simulink model "trajectory_planner"  (R2019b)
settings: Solver=FixedStepAuto  StartTime=0.0  StopTime=10.0  RelTol=1e-3
undefined symbols (not defined in the file): v
libraries: robotcorelib x1
settings Model: Creator=logan  LastModifiedBy=logan
settings OptimizationCC: DefaultParameterBehavior=Inlined  UseDivisionForNetSlopeComputation=on  GainParamInheritBuiltInType=on  UseFloatMulNetSlope=on  InlineInvariantSignals=on  PassReuseOutputArgsAs=Individual arguments  ZeroExternalMemoryAtStartup=off  ZeroInternalMemoryAtStartup=off  NoFixptDivByZeroProtection=on  EfficientFloat2IntCast=on  LifeSpan=1  OptimizeBlockOrder=speed  DifferentSizesBufferReuse=on  EfficientTunableParamExpr=on
settings DebuggingCC: ParameterTunabilityLossMsg=error
settings HardwareCC: ProdLongLongMode=on
settings SFSimCC: MATLABDynamicMemAlloc=off
settings RTWCC: SystemTargetFile=ert.tlc  TemplateMakefile=ert_default_tmf  GenerateReport=on  IncludeHyperlinkInReport=on  LaunchReport=on  TargetLang=C++  GenerateTraceInfo=on  GenerateTraceReport=on  GenerateTraceReportSl=on  GenerateTraceReportSf=on  GenerateTraceReportEml=on
settings CodeAppCC: ForceParamTrailComments=on  IgnoreCustomStorageClasses=off  OperatorAnnotations=on  SimulinkDataObjDesc=on  SFDataObjDesc=on  InsertBlockDesc=on
settings ERTTargetCC: TargetLangStandard=C++03 (ISO)  GenerateSampleERTMain=on  IncludeMdlTerminateFcn=off  CombineSignalStateStructs=on  MultiInstanceERTCode=on  CodeInterfacePackaging=C++ class  SupportComplex=off  SupportContinuousTime=on  InlinedParameterPlacement=NonHierarchical  RootIOFormat=Structure reference  ERTCustomFileTemplate=example_file_process.tlc  ERTFilePackagingFormat=CompactWithDataFile

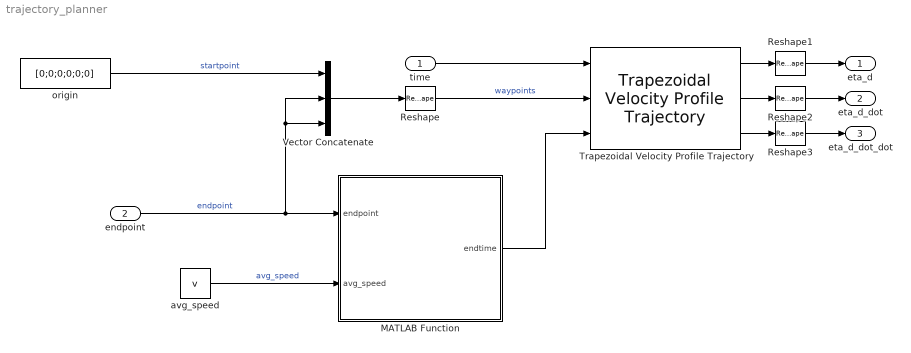
== system trajectory_planner ==
  time : Inport  PortDimensions=1
  endpoint : Inport  Port=2  PortDimensions=6
  MATLAB Function : MATLAB Function  TreatAsAtomicUnit=on
  Reshape : Reshape  OutputDimensionality=Customize  OutputDimensions=[6,3]
  Reshape1 : Reshape
  Reshape2 : Reshape
  Reshape3 : Reshape
  Trapezoidal Velocity Profile Trajectory : robotcorelib/Trapezoidal Velocity Profile Trajectory  WaypointSource=External  Waypoints=[ 0, -0.5, -1; 0, 0.5, 1 ]  NumParams=1  Parameter1=End Time  Parameter2=Peak Velocity  ParameterSource=External  PeakVelocity=[ 2; 2 ]  Acceleration=[ 1; 2 ]  EndTime=[ 1; 1 ]  AccelTime=[ 1; 2 ]  SimulateUsing=Interpreted execution
      settings: SourceProductName=Robotics System Toolbox  SourceProductBaseCode=RO
  Vector Concatenate : Concatenate  NumInputs=3
  avg_speed : Constant  Value=v
  origin : Constant  Value=[0;0;0;0;0;0]
  eta_d : Outport
  eta_d_dot : Outport  Port=2
  eta_d_dot_dot : Outport  Port=3
  wires:
  time/1 -> Trapezoidal Velocity Profile Trajectory/1
  origin/1 -> Vector Concatenate/1  "startpoint"
  Reshape2/1 -> eta_d_dot/1
  Reshape3/1 -> eta_d_dot_dot/1
  avg_speed/1 -> MATLAB Function/2(avg_speed)  "avg_speed"
  Trapezoidal Velocity Profile Trajectory/3 -> Reshape3/1
  Reshape1/1 -> eta_d/1
  Trapezoidal Velocity Profile Trajectory/2 -> Reshape2/1
  Reshape/1 -> Trapezoidal Velocity Profile Trajectory/2  "waypoints"
  Trapezoidal Velocity Profile Trajectory/1 -> Reshape1/1
  endpoint/1 -> Vector Concatenate/2, Vector Concatenate/3, MATLAB Function/1(endpoint)  "endpoint"
  MATLAB Function/1(endtime) -> Trapezoidal Velocity Profile Trajectory/3
  Vector Concatenate/1 -> Reshape/1

== matlab function trajectory_planner/MATLAB Function ==
  data: endpoint input size=6; endtime output size=1; avg_speed input
function endtime = endtime_calculation(endpoint, avg_speed)
%#codegen

% Endtime is calculated as dist from 0 to endpoint divided by avg speed
endtime = norm(endpoint)/avg_speed;

% Needed for simulation to compile (won't happen in actual use case)
if endtime <= 0
    endtime = 1;
end

end
